simulink model "ALL_JP360_DBW_V6_5_1103"  (R2022a)
settings: Solver=FixedStepAuto  StartTime=0.0  StopTime=inf  FixedStep=0.01  RelTol=1e-3  EnableMultiTasking=on
model workspace (MAT data in the model file):
  g = 9.8
undefined symbols (not defined in the file or in its folder): canChannel, delta_v_p, IPM_Line_C0, IPM_Line_C1, IPM_Line_C2, IPM_Line_C3, M, M_p, MRR_ObjDistX, MRR_ObjDistY, MRR_ObjFusionCamID, MRR_ObjFusionSig, MRR_ObjID, MRR_ObjRelVelX, MRR_ObjRelVelY, MRR_ObjType, MRR_ObjUpdFlg, none, obj_vaild, untracktime, V, videoinput
libraries: canfdmsglib x230, canfdlib x76, slpidlib x24, simulink x18, dspstat3 x14, ctrlSharedLib x1, simulink_extras x1, imaqlib x1, realtime_pacer_lib x1, dspvision x1, visionsinks x1
(part 12 of 55)

== system ALL_JP360_DBW_V6_5_1103/MsgFromCAN/CCAN_ADCU_MsgFromCAN/CCAN_ADCU_SWM_Body_0x31A ==
  CCAN_ADCU_SWM_Body_0x31AFromInData : Inport  OutDataTypeStr=Bus:CAN_FD_MESSAGE_BUS
  Bus Creator : BusCreator  Inputs=28  OutDataTypeStr=Bus:CCAN_ADCU_SWM_Body_0x31A  NonVirtualBus=on
  CAN FD Unpack : canfdmsglib/CAN FD Unpack  CANdbFile=HiFire_JPT360_CCAN_Matrix_CAN_V1.72_VP_ADCU.dbc  MsgList=(none)  MsgName=SWM_Body_0x31A  ProtocolMode=CAN FD  MsgIDType=Standard (11-bit identifier)  MsgIdentifier=794  MsgLength=8  SignalInfo={'Checksum_0x31A','56','8','BE','unsigned','Standard','0','1','0','0','255';'RollingCounter_0x31A','48','4','BE','unsigned','Standard','0','1','0','0','15';'SWM_FWasherSts','4','2','BE','unsigned','Standard','0','1','0','0','3';'SWM_FlashLightSts','8','2','BE','unsigned','Standard','0','1','0','0','3';'SWM_FrontFogLight','18','2','BE','unsigned','Standard','0','1','0','0','3';'SWM_FrontWipingMode','10','3','BE','unsigned','Standard','0','1','0','0','7';'SWM_HeadLamp','29','3','BE','unsigned','Standard','0','1','0','0','3';'SWM_HighBeam','0','2','BE','unsigned','Standard','0','1','0','0','3';'SWM_LampLimpHomeSts','3','1','BE','unsigned','Standard','0','1','0','0','1';'SWM_Menu_Confirm','54','2','BE','unsigned','Standard','0','1','0','0','3';'SWM_Menu_Down','44','2','BE','unsigned','Standard','0','1','0','0','3';'SWM_Menu_Left','42','2','BE','unsigned','Standard','0','1','0','0','3';'SWM_Menu_Return','52','2','BE','unsigned','Standard','0','1','0','0','3';'SWM_Menu_Right','40','2','BE','unsigned','Standard','0','1','0','0','3';'SWM_Menu_Up','46','2','BE','unsigned','Standard','0','1','0','0','3';'SWM_Mute','38','2','BE','unsigned','Standard','0','1','0','0','3';'SWM_Next_Song','32','2','BE','unsigned','Standard','0','1','0','0','3';'SWM_Phone','36','2','BE','unsigned','Standard','0','1','0','0','3';'SWM_Previous_Song','34','2','BE','unsigned','Standard','0','1','0','0','3';'SWM_RWasherSts','6','2','BE','unsigned','Standard','0','1','0','0','3';'SWM_RearFogLight','16','2','BE','unsigned','Standard','0','1','0','0','3';'SWM_RearWipingMode','20','2','BE','unsigned','Standard','0','1','0','0','3';'SWM_TurnIndicationAct','22','2','BE','unsigned','Standard','0','1','0','0','3';'SWM_VOL_Minus','26','2','BE','unsigned','Standard','0','1','0','0','3';'SWM_VOL_Plus','24','2','BE','unsigned','Standard','0','1','0','0','3';'SWM_WasherLimpHomeSts','2','1','BE','unsigned','Standard','0','1','0','0','1';'SWM_Wechat','28','1','BE','unsigned','Standard','0','1','0','0','1';'SWM_WipingInterval_Sensitvity','13','3','BE','unsigned','Standard','0','1','0','0','7'}  IDPort=off  TimestampPort=off  ErrorPort=off  RemotePort=off  LengthPort=off  StatusPort=off  BRSPort=off  ESIPort=off  DLCPort=off  ApplyMinMax=off
      settings: SourceProductBaseCode=XP,ME,VN  DataFormat=CANdb specified signals
  Data Type Conversion1 : DataTypeConversion  OutDataTypeStr=uint8  SaturateOnIntegerOverflow=off  RndMeth=Floor
  Data Type Conversion{2..8,10..25,28} (24 alike) : DataTypeConversion  OutDataTypeStr=int8  SaturateOnIntegerOverflow=off  RndMeth=Floor
  Data Type Conversion26 : DataTypeConversion  OutDataTypeStr=boolean  SaturateOnIntegerOverflow=off  RndMeth=Floor
  Data Type Conversion27 : DataTypeConversion  OutDataTypeStr=boolean  SaturateOnIntegerOverflow=off  RndMeth=Floor
  Data Type Conversion9 : DataTypeConversion  OutDataTypeStr=boolean  SaturateOnIntegerOverflow=off  RndMeth=Floor
  CCAN_ADCU_SWM_Body_0x31AFromOutData : Outport  OutDataTypeStr=Bus:CCAN_ADCU_SWM_Body_0x31A
  wires:
  CAN FD Unpack/1 -> Data Type Conversion1/1
  CAN FD Unpack/2 -> Data Type Conversion2/1
  CAN FD Unpack/3 -> Data Type Conversion3/1
  CAN FD Unpack/4 -> Data Type Conversion4/1
  CAN FD Unpack/5 -> Data Type Conversion5/1
  CAN FD Unpack/6 -> Data Type Conversion6/1
  CAN FD Unpack/7 -> Data Type Conversion7/1
  CAN FD Unpack/8 -> Data Type Conversion8/1
  CAN FD Unpack/9 -> Data Type Conversion9/1
  CAN FD Unpack/10 -> Data Type Conversion10/1
  CAN FD Unpack/11 -> Data Type Conversion11/1
  CAN FD Unpack/12 -> Data Type Conversion12/1
  CAN FD Unpack/13 -> Data Type Conversion13/1
  CAN FD Unpack/14 -> Data Type Conversion14/1
  CAN FD Unpack/15 -> Data Type Conversion15/1
  CAN FD Unpack/16 -> Data Type Conversion16/1
  CAN FD Unpack/17 -> Data Type Conversion17/1
  CAN FD Unpack/18 -> Data Type Conversion18/1
  CAN FD Unpack/19 -> Data Type Conversion19/1
  CAN FD Unpack/20 -> Data Type Conversion20/1
  CAN FD Unpack/21 -> Data Type Conversion21/1
  CAN FD Unpack/22 -> Data Type Conversion22/1
  CAN FD Unpack/23 -> Data Type Conversion23/1
  CAN FD Unpack/24 -> Data Type Conversion24/1
  CAN FD Unpack/25 -> Data Type Conversion25/1
  CAN FD Unpack/26 -> Data Type Conversion26/1
  CAN FD Unpack/27 -> Data Type Conversion27/1
  CAN FD Unpack/28 -> Data Type Conversion28/1
  Data Type Conversion1/1 -> Bus Creator/1  "Checksum_0x31A"
  Data Type Conversion2/1 -> Bus Creator/2  "RollingCounter_0x31A"
  Data Type Conversion3/1 -> Bus Creator/3  "SWM_FWasherSts"
  Data Type Conversion4/1 -> Bus Creator/4  "SWM_FlashLightSts"
  Data Type Conversion5/1 -> Bus Creator/5  "SWM_FrontFogLight"
  Data Type Conversion6/1 -> Bus Creator/6  "SWM_FrontWipingMode"
  Data Type Conversion7/1 -> Bus Creator/7  "SWM_HeadLamp"
  Data Type Conversion8/1 -> Bus Creator/8  "SWM_HighBeam"
  Data Type Conversion9/1 -> Bus Creator/9  "SWM_LampLimpHomeSts"
  Data Type Conversion10/1 -> Bus Creator/10  "SWM_Menu_Confirm"
  Data Type Conversion11/1 -> Bus Creator/11  "SWM_Menu_Down"
  Data Type Conversion12/1 -> Bus Creator/12  "SWM_Menu_Left"
  Data Type Conversion13/1 -> Bus Creator/13  "SWM_Menu_Return"
  Data Type Conversion14/1 -> Bus Creator/14  "SWM_Menu_Right"
  Data Type Conversion15/1 -> Bus Creator/15  "SWM_Menu_Up"
  Data Type Conversion16/1 -> Bus Creator/16  "SWM_Mute"
  Data Type Conversion17/1 -> Bus Creator/17  "SWM_Next_Song"
  Data Type Conversion18/1 -> Bus Creator/18  "SWM_Phone"
  Data Type Conversion19/1 -> Bus Creator/19  "SWM_Previous_Song"
  Data Type Conversion20/1 -> Bus Creator/20  "SWM_RWasherSts"
  Data Type Conversion21/1 -> Bus Creator/21  "SWM_RearFogLight"
  Data Type Conversion22/1 -> Bus Creator/22  "SWM_RearWipingMode"
  Data Type Conversion23/1 -> Bus Creator/23  "SWM_TurnIndicationAct"
  Data Type Conversion24/1 -> Bus Creator/24  "SWM_VOL_Minus"
  Data Type Conversion25/1 -> Bus Creator/25  "SWM_VOL_Plus"
  Data Type Conversion26/1 -> Bus Creator/26  "SWM_WasherLimpHomeSts"
  Data Type Conversion27/1 -> Bus Creator/27  "SWM_Wechat"
  Data Type Conversion28/1 -> Bus Creator/28  "SWM_WipingInterval_Sensitvity"
  Bus Creator/1 -> CCAN_ADCU_SWM_Body_0x31AFromOutData/1  "CCAN_ADCU_SWM_Body_0x31AFromOutData"
  CCAN_ADCU_SWM_Body_0x31AFromInData/1 -> CAN FD Unpack/1  "CCAN_ADCU_SWM_Body_0x31AFromInData"

== system ALL_JP360_DBW_V6_5_1103/MsgFromCAN/CCAN_ADCU_MsgFromCAN/CCAN_ADCU_SWM_MRR_0x31B ==
  CCAN_ADCU_SWM_MRR_0x31BFromInData : Inport  OutDataTypeStr=Bus:CAN_FD_MESSAGE_BUS
  Bus Creator : BusCreator  Inputs=22  OutDataTypeStr=Bus:CCAN_ADCU_SWM_MRR_0x31B  NonVirtualBus=on
  CAN FD Unpack : canfdmsglib/CAN FD Unpack  CANdbFile=HiFire_JPT360_CCAN_Matrix_CAN_V1.72_VP_ADCU.dbc  MsgList=(none)  MsgName=SWM_MRR_0x31B  ProtocolMode=CAN FD  MsgIDType=Standard (11-bit identifier)  MsgIdentifier=795  MsgLength=8  SignalInfo={'BCM_CCO_Switch','20','1','BE','unsigned','Standard','0','1','0','0','1';'BCM_TAB_Switch','19','1','BE','unsigned','Standard','0','1','0','0','1';'Checksum_0x31B','56','8','BE','unsigned','Standard','0','1','0','0','255';'RollingCounter_0x31B','48','4','BE','unsigned','Standard','0','1','0','0','15';'SWM_ACCDeactivate','3','1','BE','unsigned','Standard','0','1','0','0','1';'SWM_ACCLimpHomeSts','11','1','BE','unsigned','Standard','0','1','0','0','1';'SWM_ACCResume','4','1','BE','unsigned','Standard','0','1','0','0','1';'SWM_ACCResume_Qt','7','1','BE','unsigned','Standard','0','1','0','0','1';'SWM_ACCSet','5','1','BE','unsigned','Standard','0','1','0','0','1';'SWM_ACCSwitch','12','1','BE','unsigned','Standard','0','1','0','0','1';'SWM_ACCtauGapSetMinus','15','1','BE','unsigned','Standard','0','1','0','0','1';'SWM_ACCtauGapSetPlus','0','1','BE','unsigned','Standard','0','1','0','0','1';'SWM_ACCvSetMinus','1','1','BE','unsigned','Standard','0','1','0','0','1';'SWM_ACCvSetPlus','2','1','BE','unsigned','Standard','0','1','0','0','1';'SWM_CCEnableSwitch','6','1','BE','unsigned','Standard','0','1','0','0','1';'SWM_ICorIVI','21','1','BE','unsigned','Standard','0','1','0','0','1';'SWM_LaneAssistSwitch','14','1','BE','unsigned','Standard','0','1','0','0','1';'SWM_MyButton','22','1','BE','unsigned','Standard','0','1','0','0','1';'SWM_ShiftPadFlt','23','1','BE','unsigned','Standard','0','1','0','0','1';'SWM_ShiftPadReqDown','9','1','BE','unsigned','Standard','0','1','0','0','1';'SWM_ShiftPadReqUp','10','1','BE','unsigned','Standard','0','1','0','0','1';'SWM_TJASwitch','8','1','BE','unsigned','Standard','0','1','0','0','1'}  IDPort=off  TimestampPort=off  ErrorPort=off  RemotePort=off  LengthPort=off  StatusPort=off  BRSPort=off  ESIPort=off  DLCPort=off  ApplyMinMax=off
      settings: SourceProductBaseCode=XP,ME,VN  DataFormat=CANdb specified signals
  Data Type Conversion{1..2,5..22} (20 alike) : DataTypeConversion  OutDataTypeStr=boolean  SaturateOnIntegerOverflow=off  RndMeth=Floor
  Data Type Conversion3 : DataTypeConversion  OutDataTypeStr=uint8  SaturateOnIntegerOverflow=off  RndMeth=Floor
  Data Type Conversion4 : DataTypeConversion  OutDataTypeStr=int8  SaturateOnIntegerOverflow=off  RndMeth=Floor
  CCAN_ADCU_SWM_MRR_0x31BFromOutData : Outport  OutDataTypeStr=Bus:CCAN_ADCU_SWM_MRR_0x31B
  wires:
  CAN FD Unpack/1 -> Data Type Conversion1/1
  CAN FD Unpack/2 -> Data Type Conversion2/1
  CAN FD Unpack/3 -> Data Type Conversion3/1
  CAN FD Unpack/4 -> Data Type Conversion4/1
  CAN FD Unpack/5 -> Data Type Conversion5/1
  CAN FD Unpack/6 -> Data Type Conversion6/1
  CAN FD Unpack/7 -> Data Type Conversion7/1
  CAN FD Unpack/8 -> Data Type Conversion8/1
  CAN FD Unpack/9 -> Data Type Conversion9/1
  CAN FD Unpack/10 -> Data Type Conversion10/1
  CAN FD Unpack/11 -> Data Type Conversion11/1
  CAN FD Unpack/12 -> Data Type Conversion12/1
  CAN FD Unpack/13 -> Data Type Conversion13/1
  CAN FD Unpack/14 -> Data Type Conversion14/1
  CAN FD Unpack/15 -> Data Type Conversion15/1
  CAN FD Unpack/16 -> Data Type Conversion16/1
  CAN FD Unpack/17 -> Data Type Conversion17/1
  CAN FD Unpack/18 -> Data Type Conversion18/1
  CAN FD Unpack/19 -> Data Type Conversion19/1
  CAN FD Unpack/20 -> Data Type Conversion20/1
  CAN FD Unpack/21 -> Data Type Conversion21/1
  CAN FD Unpack/22 -> Data Type Conversion22/1
  Data Type Conversion1/1 -> Bus Creator/1  "BCM_CCO_Switch"
  Data Type Conversion2/1 -> Bus Creator/2  "BCM_TAB_Switch"
  Data Type Conversion3/1 -> Bus Creator/3  "Checksum_0x31B"
  Data Type Conversion4/1 -> Bus Creator/4  "RollingCounter_0x31B"
  Data Type Conversion5/1 -> Bus Creator/5  "SWM_ACCDeactivate"
  Data Type Conversion6/1 -> Bus Creator/6  "SWM_ACCLimpHomeSts"
  Data Type Conversion7/1 -> Bus Creator/7  "SWM_ACCResume"
  Data Type Conversion8/1 -> Bus Creator/8  "SWM_ACCResume_Qt"
  Data Type Conversion9/1 -> Bus Creator/9  "SWM_ACCSet"
  Data Type Conversion10/1 -> Bus Creator/10  "SWM_ACCSwitch"
  Data Type Conversion11/1 -> Bus Creator/11  "SWM_ACCtauGapSetMinus"
  Data Type Conversion12/1 -> Bus Creator/12  "SWM_ACCtauGapSetPlus"
  Data Type Conversion13/1 -> Bus Creator/13  "SWM_ACCvSetMinus"
  Data Type Conversion14/1 -> Bus Creator/14  "SWM_ACCvSetPlus"
  Data Type Conversion15/1 -> Bus Creator/15  "SWM_CCEnableSwitch"
  Data Type Conversion16/1 -> Bus Creator/16  "SWM_ICorIVI"
  Data Type Conversion17/1 -> Bus Creator/17  "SWM_LaneAssistSwitch"
  Data Type Conversion18/1 -> Bus Creator/18  "SWM_MyButton"
  Data Type Conversion19/1 -> Bus Creator/19  "SWM_ShiftPadFlt"
  Data Type Conversion20/1 -> Bus Creator/20  "SWM_ShiftPadReqDown"
  Data Type Conversion21/1 -> Bus Creator/21  "SWM_ShiftPadReqUp"
  Data Type Conversion22/1 -> Bus Creator/22  "SWM_TJASwitch"
  Bus Creator/1 -> CCAN_ADCU_SWM_MRR_0x31BFromOutData/1  "CCAN_ADCU_SWM_MRR_0x31BFromOutData"
  CCAN_ADCU_SWM_MRR_0x31BFromInData/1 -> CAN FD Unpack/1  "CCAN_ADCU_SWM_MRR_0x31BFromInData"

== system ALL_JP360_DBW_V6_5_1103/MsgFromCAN/CCAN_ADCU_MsgFromCAN/CCAN_ADCU_Tester_DiagFuncReq ==
  CCAN_ADCU_Tester_DiagFuncReqFromInData : Inport  OutDataTypeStr=Bus:CAN_FD_MESSAGE_BUS
  Bus Creator : BusCreator  Inputs=1  OutDataTypeStr=Bus:CCAN_ADCU_Tester_DiagFuncReq  NonVirtualBus=on
  CAN FD Unpack : canfdmsglib/CAN FD Unpack  CANdbFile=HiFire_JPT360_CCAN_Matrix_CAN_V1.72_VP_ADCU.dbc  MsgList=(none)  MsgName=Tester_DiagFuncReq  ProtocolMode=CAN FD  MsgIDType=Standard (11-bit identifier)  MsgIdentifier=2015  MsgLength=8  SignalInfo={'DiagFuncReq','56','64','BE','unsigned','Standard','0','1','0','0','1.84467440737095e+19'}  IDPort=off  TimestampPort=off  ErrorPort=off  RemotePort=off  LengthPort=off  StatusPort=off  BRSPort=off  ESIPort=off  DLCPort=off  ApplyMinMax=off
      settings: SourceProductBaseCode=XP,ME,VN  DataFormat=CANdb specified signals
  Data Type Conversion1 : DataTypeConversion  OutDataTypeStr=uint64  SaturateOnIntegerOverflow=off  RndMeth=Floor
  CCAN_ADCU_Tester_DiagFuncReqFromOutData : Outport  OutDataTypeStr=Bus:CCAN_ADCU_Tester_DiagFuncReq
  wires:
  Data Type Conversion1/1 -> Bus Creator/1  "DiagFuncReq"
  Bus Creator/1 -> CCAN_ADCU_Tester_DiagFuncReqFromOutData/1  "CCAN_ADCU_Tester_DiagFuncReqFromOutData"
  CCAN_ADCU_Tester_DiagFuncReqFromInData/1 -> CAN FD Unpack/1  "CCAN_ADCU_Tester_DiagFuncReqFromInData"

== system ALL_JP360_DBW_V6_5_1103/MsgFromCAN/CCAN_ADCU_MsgFromCAN/CCAN_ADCU_Tester_DiagReqToADCU ==
  CCAN_ADCU_Tester_DiagReqToADCUFromInData : Inport  OutDataTypeStr=Bus:CAN_FD_MESSAGE_BUS
  Bus Creator : BusCreator  Inputs=1  OutDataTypeStr=Bus:CCAN_ADCU_Tester_DiagReqToADCU  NonVirtualBus=on
  CAN FD Unpack : canfdmsglib/CAN FD Unpack  CANdbFile=HiFire_JPT360_CCAN_Matrix_CAN_V1.72_VP_ADCU.dbc  MsgList=(none)  MsgName=Tester_DiagReqToADCU  ProtocolMode=CAN FD  MsgIDType=Standard (11-bit identifier)  MsgIdentifier=1809  MsgLength=8  SignalInfo={'DiagPhysReqToADCU','56','64','BE','unsigned','Standard','0','1','0','0','1.84467440737095e+19'}  IDPort=off  TimestampPort=off  ErrorPort=off  RemotePort=off  LengthPort=off  StatusPort=off  BRSPort=off  ESIPort=off  DLCPort=off  ApplyMinMax=off
      settings: SourceProductBaseCode=XP,ME,VN  DataFormat=CANdb specified signals
  Data Type Conversion1 : DataTypeConversion  OutDataTypeStr=uint64  SaturateOnIntegerOverflow=off  RndMeth=Floor
  CCAN_ADCU_Tester_DiagReqToADCUFromOutData : Outport  OutDataTypeStr=Bus:CCAN_ADCU_Tester_DiagReqToADCU
  wires:
  Data Type Conversion1/1 -> Bus Creator/1  "DiagPhysReqToADCU"
  Bus Creator/1 -> CCAN_ADCU_Tester_DiagReqToADCUFromOutData/1  "CCAN_ADCU_Tester_DiagReqToADCUFromOutData"
  CCAN_ADCU_Tester_DiagReqToADCUFromInData/1 -> CAN FD Unpack/1  "CCAN_ADCU_Tester_DiagReqToADCUFromInData"

== system ALL_JP360_DBW_V6_5_1103/MsgFromCAN/CCAN_GW_MsgFromCAN/CCAN_GW_ABS_Sts_0x221 ==
  CCAN_GW_ABS_Sts_0x221FromInData : Inport  OutDataTypeStr=Bus:CAN_FD_MESSAGE_BUS
  Bus Creator : BusCreator  Inputs=12  OutDataTypeStr=Bus:CCAN_GW_ABS_Sts_0x221  NonVirtualBus=on
  CAN FD Unpack : canfdmsglib/CAN FD Unpack  CANdbFile=HiFire_JPT360_CCAN_Matrix_CAN_V1.72_VP_ADCU.dbc  MsgList=(none)  MsgName=ABS_Sts_0x221  ProtocolMode=CAN FD  MsgIDType=Standard (11-bit identifier)  MsgIdentifier=545  MsgLength=8  SignalInfo={'ABS_AbsCtrlActv','39','1','BE','unsigned','Standard','0','1','0','0','1';'ABS_AbsFlgFlt','38','1','BE','unsigned','Standard','0','1','0','0','1';'ABS_EbdFlgFlt','37','1','BE','unsigned','Standard','0','1','0','0','1';'ABS_VehSpdDirection','36','1','BE','unsigned','Standard','0','1','0','0','1';'ABS_VehSpdLgt','40','12','BE','unsigned','Standard','0','0.05625','0','0','230.2875';'ABS_VehSpdLgtStatus','54','2','BE','unsigned','Standard','0','1','0','0','2';'ABS_WhlMilgFrntLe','8','16','BE','unsigned','Standard','0','1','0','0','65535';'ABS_WhlMilgFrntLeStatus','52','1','BE','unsigned','Standard','0','1','0','0','1';'ABS_WhlMilgFrntRi','24','16','BE','unsigned','Standard','0','1','0','0','65535';'ABS_WhlMilgFrntRiStatus','53','1','BE','unsigned','Standard','0','1','0','0','1';'Checksum_0x221','56','8','BE','unsigned','Standard','0','1','0','0','255';'RollingCounter_0x221','48','4','BE','unsigned','Standard','0','1','0','0','15'}  IDPort=off  TimestampPort=off  ErrorPort=off  RemotePort=off  LengthPort=off  StatusPort=off  BRSPort=off  ESIPort=off  DLCPort=off  ApplyMinMax=off
      settings: SourceProductBaseCode=XP,ME,VN  DataFormat=CANdb specified signals
  Data Type Conversion{1..4,8,10} (6 alike) : DataTypeConversion  OutDataTypeStr=boolean  SaturateOnIntegerOverflow=off  RndMeth=Floor
  Data Type Conversion11 : DataTypeConversion  OutDataTypeStr=uint8  SaturateOnIntegerOverflow=off  RndMeth=Floor
  Data Type Conversion12 : DataTypeConversion  OutDataTypeStr=int8  SaturateOnIntegerOverflow=off  RndMeth=Floor
  Data Type Conversion5 : DataTypeConversion  OutDataTypeStr=single  SaturateOnIntegerOverflow=off  RndMeth=Floor
  Data Type Conversion6 : DataTypeConversion  OutDataTypeStr=int8  SaturateOnIntegerOverflow=off  RndMeth=Floor
  Data Type Conversion7 : DataTypeConversion  OutDataTypeStr=uint16  SaturateOnIntegerOverflow=off  RndMeth=Floor
  Data Type Conversion9 : DataTypeConversion  OutDataTypeStr=uint16  SaturateOnIntegerOverflow=off  RndMeth=Floor
  CCAN_GW_ABS_Sts_0x221FromOutData : Outport  OutDataTypeStr=Bus:CCAN_GW_ABS_Sts_0x221
  wires:
  CAN FD Unpack/1 -> Data Type Conversion1/1
  CAN FD Unpack/2 -> Data Type Conversion2/1
  CAN FD Unpack/3 -> Data Type Conversion3/1
  CAN FD Unpack/4 -> Data Type Conversion4/1
  CAN FD Unpack/5 -> Data Type Conversion5/1
  CAN FD Unpack/6 -> Data Type Conversion6/1
  CAN FD Unpack/7 -> Data Type Conversion7/1
  CAN FD Unpack/8 -> Data Type Conversion8/1
  CAN FD Unpack/9 -> Data Type Conversion9/1
  CAN FD Unpack/10 -> Data Type Conversion10/1
  CAN FD Unpack/11 -> Data Type Conversion11/1
  CAN FD Unpack/12 -> Data Type Conversion12/1
  Data Type Conversion1/1 -> Bus Creator/1  "ABS_AbsCtrlActv"
  Data Type Conversion2/1 -> Bus Creator/2  "ABS_AbsFlgFlt"
  Data Type Conversion3/1 -> Bus Creator/3  "ABS_EbdFlgFlt"
  Data Type Conversion4/1 -> Bus Creator/4  "ABS_VehSpdDirection"
  Data Type Conversion5/1 -> Bus Creator/5  "ABS_VehSpdLgt"
  Data Type Conversion6/1 -> Bus Creator/6  "ABS_VehSpdLgtStatus"
  Data Type Conversion7/1 -> Bus Creator/7  "ABS_WhlMilgFrntLe"
  Data Type Conversion8/1 -> Bus Creator/8  "ABS_WhlMilgFrntLeStatus"
  Data Type Conversion9/1 -> Bus Creator/9  "ABS_WhlMilgFrntRi"
  Data Type Conversion10/1 -> Bus Creator/10  "ABS_WhlMilgFrntRiStatus"
  Data Type Conversion11/1 -> Bus Creator/11  "Checksum_0x221"
  Data Type Conversion12/1 -> Bus Creator/12  "RollingCounter_0x221"
  Bus Creator/1 -> CCAN_GW_ABS_Sts_0x221FromOutData/1  "CCAN_GW_ABS_Sts_0x221FromOutData"
  CCAN_GW_ABS_Sts_0x221FromInData/1 -> CAN FD Unpack/1  "CCAN_GW_ABS_Sts_0x221FromInData"

== system ALL_JP360_DBW_V6_5_1103/MsgFromCAN/CCAN_GW_MsgFromCAN/CCAN_GW_ABS_Vspeed_0x601 ==
  CCAN_GW_ABS_Vspeed_0x601FromInData : Inport  OutDataTypeStr=Bus:CAN_FD_MESSAGE_BUS
  Bus Creator : BusCreator  Inputs=2  OutDataTypeStr=Bus:CCAN_GW_ABS_Vspeed_0x601  NonVirtualBus=on
  CAN FD Unpack : canfdmsglib/CAN FD Unpack  CANdbFile=HiFire_JPT360_CCAN_Matrix_CAN_V1.72_VP_ADCU.dbc  MsgList=(none)  MsgName=ABS_Vspeed_0x601  ProtocolMode=CAN FD  MsgIDType=Standard (11-bit identifier)  MsgIdentifier=1537  MsgLength=8  SignalInfo={'ABS_VehSpd','8','16','BE','unsigned','Standard','0','0.0039062','0','0','250.996';'ABS_VehSpd_GB1','24','16','BE','unsigned','Standard','0','0.1','0','0','220'}  IDPort=off  TimestampPort=off  ErrorPort=off  RemotePort=off  LengthPort=off  StatusPort=off  BRSPort=off  ESIPort=off  DLCPort=off  ApplyMinMax=off
      settings: SourceProductBaseCode=XP,ME,VN  DataFormat=CANdb specified signals
  Data Type Conversion1 : DataTypeConversion  OutDataTypeStr=single  SaturateOnIntegerOverflow=off  RndMeth=Floor
  Data Type Conversion2 : DataTypeConversion  OutDataTypeStr=single  SaturateOnIntegerOverflow=off  RndMeth=Floor
  CCAN_GW_ABS_Vspeed_0x601FromOutData : Outport  OutDataTypeStr=Bus:CCAN_GW_ABS_Vspeed_0x601
  wires:
  CAN FD Unpack/1 -> Data Type Conversion1/1
  CAN FD Unpack/2 -> Data Type Conversion2/1
  Data Type Conversion1/1 -> Bus Creator/1  "ABS_VehSpd"
  Data Type Conversion2/1 -> Bus Creator/2  "ABS_VehSpd_GB1"
  Bus Creator/1 -> CCAN_GW_ABS_Vspeed_0x601FromOutData/1  "CCAN_GW_ABS_Vspeed_0x601FromOutData"
  CCAN_GW_ABS_Vspeed_0x601FromInData/1 -> CAN FD Unpack/1  "CCAN_GW_ABS_Vspeed_0x601FromInData"

== system ALL_JP360_DBW_V6_5_1103/MsgFromCAN/CCAN_GW_MsgFromCAN/CCAN_GW_ABS_WhlSpd_0x211 ==
  CCAN_GW_ABS_WhlSpd_0x211FromInData : Inport  OutDataTypeStr=Bus:CAN_FD_MESSAGE_BUS
  Bus Creator : BusCreator  Inputs=10  OutDataTypeStr=Bus:CCAN_GW_ABS_WhlSpd_0x211  NonVirtualBus=on
  CAN FD Unpack : canfdmsglib/CAN FD Unpack  CANdbFile=HiFire_JPT360_CCAN_Matrix_CAN_V1.72_VP_ADCU.dbc  MsgList=(none)  MsgName=ABS_WhlSpd_0x211  ProtocolMode=CAN FD  MsgIDType=Standard (11-bit identifier)  MsgIdentifier=529  MsgLength=8  SignalInfo={'ABS_WhlSpdFrntLe','12','12','BE','unsigned','Standard','0','0.05625','0','0','230.2875';'ABS_WhlSpdFrntLeStatus','55','1','BE','unsigned','Standard','0','1','0','0','1';'ABS_WhlSpdFrntRi','16','12','BE','unsigned','Standard','0','0.05625','0','0','230.2875';'ABS_WhlSpdFrntRiStatus','54','1','BE','unsigned','Standard','0','1','0','0','1';'ABS_WhlSpdReLe','36','12','BE','unsigned','Standard','0','0.05625','0','0','230.2875';'ABS_WhlSpdReLeStatus','53','1','BE','unsigned','Standard','0','1','0','0','1';'ABS_WhlSpdReRi','40','12','BE','unsigned','Standard','0','0.05625','0','0','230.2875';'ABS_WhlSpdReRiStatus','52','1','BE','unsigned','Standard','0','1','0','0','1';'Checksum_0x211','56','8','BE','unsigned','Standard','0','1','0','0','255';'RollingCounter_0x211','48','4','BE','unsigned','Standard','0','1','0','0','15'}  IDPort=off  TimestampPort=off  ErrorPort=off  RemotePort=off  LengthPort=off  StatusPort=off  BRSPort=off  ESIPort=off  DLCPort=off  ApplyMinMax=off
      settings: SourceProductBaseCode=XP,ME,VN  DataFormat=CANdb specified signals
  Data Type Conversion{1,3,5,7} (4 alike) : DataTypeConversion  OutDataTypeStr=single  SaturateOnIntegerOverflow=off  RndMeth=Floor
  Data Type Conversion10 : DataTypeConversion  OutDataTypeStr=int8  SaturateOnIntegerOverflow=off  RndMeth=Floor
  Data Type Conversion{2,4,6,8} (4 alike) : DataTypeConversion  OutDataTypeStr=boolean  SaturateOnIntegerOverflow=off  RndMeth=Floor
  Data Type Conversion9 : DataTypeConversion  OutDataTypeStr=uint8  SaturateOnIntegerOverflow=off  RndMeth=Floor
  CCAN_GW_ABS_WhlSpd_0x211FromOutData : Outport  OutDataTypeStr=Bus:CCAN_GW_ABS_WhlSpd_0x211
  wires:
  CAN FD Unpack/1 -> Data Type Conversion1/1
  CAN FD Unpack/2 -> Data Type Conversion2/1
  CAN FD Unpack/3 -> Data Type Conversion3/1
  CAN FD Unpack/4 -> Data Type Conversion4/1
  CAN FD Unpack/5 -> Data Type Conversion5/1
  CAN FD Unpack/6 -> Data Type Conversion6/1
  CAN FD Unpack/7 -> Data Type Conversion7/1
  CAN FD Unpack/8 -> Data Type Conversion8/1
  CAN FD Unpack/9 -> Data Type Conversion9/1
  CAN FD Unpack/10 -> Data Type Conversion10/1
  Data Type Conversion1/1 -> Bus Creator/1  "ABS_WhlSpdFrntLe"
  Data Type Conversion2/1 -> Bus Creator/2  "ABS_WhlSpdFrntLeStatus"
  Data Type Conversion3/1 -> Bus Creator/3  "ABS_WhlSpdFrntRi"
  Data Type Conversion4/1 -> Bus Creator/4  "ABS_WhlSpdFrntRiStatus"
  Data Type Conversion5/1 -> Bus Creator/5  "ABS_WhlSpdReLe"
  Data Type Conversion6/1 -> Bus Creator/6  "ABS_WhlSpdReLeStatus"
  Data Type Conversion7/1 -> Bus Creator/7  "ABS_WhlSpdReRi"
  Data Type Conversion8/1 -> Bus Creator/8  "ABS_WhlSpdReRiStatus"
  Data Type Conversion9/1 -> Bus Creator/9  "Checksum_0x211"
  Data Type Conversion10/1 -> Bus Creator/10  "RollingCounter_0x211"
  Bus Creator/1 -> CCAN_GW_ABS_WhlSpd_0x211FromOutData/1  "CCAN_GW_ABS_WhlSpd_0x211FromOutData"
  CCAN_GW_ABS_WhlSpd_0x211FromInData/1 -> CAN FD Unpack/1  "CCAN_GW_ABS_WhlSpd_0x211FromInData"

== system ALL_JP360_DBW_V6_5_1103/MsgFromCAN/CCAN_GW_MsgFromCAN/CCAN_GW_ADCU_0x538 ==
  CCAN_GW_ADCU_0x538FromInData : Inport  OutDataTypeStr=Bus:CAN_FD_MESSAGE_BUS
  Bus Creator : BusCreator  Inputs=2  OutDataTypeStr=Bus:CCAN_GW_ADCU_0x538  NonVirtualBus=on
  CAN FD Unpack : canfdmsglib/CAN FD Unpack  CANdbFile=HiFire_JPT360_CCAN_Matrix_CAN_V1.72_VP_ADCU.dbc  MsgList=(none)  MsgName=ADCU_0x538  ProtocolMode=CAN FD  MsgIDType=Standard (11-bit identifier)  MsgIdentifier=1336  MsgLength=8  SignalInfo={'ADCU_state','6','2','BE','unsigned','Standard','0','1','0','0','3';'BSD_FCTB_State','0','1','BE','unsigned','Standard','0','1','0','0','1'}  IDPort=off  TimestampPort=off  ErrorPort=off  RemotePort=off  LengthPort=off  StatusPort=off  BRSPort=off  ESIPort=off  DLCPort=off  ApplyMinMax=off
      settings: SourceProductBaseCode=XP,ME,VN  DataFormat=CANdb specified signals
  Data Type Conversion1 : DataTypeConversion  OutDataTypeStr=int8  SaturateOnIntegerOverflow=off  RndMeth=Floor
  Data Type Conversion2 : DataTypeConversion  OutDataTypeStr=boolean  SaturateOnIntegerOverflow=off  RndMeth=Floor
  CCAN_GW_ADCU_0x538FromOutData : Outport  OutDataTypeStr=Bus:CCAN_GW_ADCU_0x538
  wires:
  CAN FD Unpack/1 -> Data Type Conversion1/1
  CAN FD Unpack/2 -> Data Type Conversion2/1
  Data Type Conversion1/1 -> Bus Creator/1  "ADCU_state"
  Data Type Conversion2/1 -> Bus Creator/2  "BSD_FCTB_State"
  Bus Creator/1 -> CCAN_GW_ADCU_0x538FromOutData/1  "CCAN_GW_ADCU_0x538FromOutData"
  CCAN_GW_ADCU_0x538FromInData/1 -> CAN FD Unpack/1  "CCAN_GW_ADCU_0x538FromInData"

== system ALL_JP360_DBW_V6_5_1103/MsgFromCAN/CCAN_GW_MsgFromCAN/CCAN_GW_ADCU_CanTSyn_0x570 ==
  CCAN_GW_ADCU_CanTSyn_0x570FromInData : Inport  OutDataTypeStr=Bus:CAN_FD_MESSAGE_BUS
  Bus Creator : BusCreator  Inputs=1  OutDataTypeStr=Bus:CCAN_GW_ADCU_CanTSyn_0x570  NonVirtualBus=on
  CAN FD Unpack : canfdmsglib/CAN FD Unpack  CANdbFile=HiFire_JPT360_CCAN_Matrix_CAN_V1.72_VP_ADCU.dbc  MsgList=(none)  MsgName=ADCU_CanTSyn_0x570  ProtocolMode=CAN FD  MsgIDType=Standard (11-bit identifier)  MsgIdentifier=1392  MsgLength=8  SignalInfo={'CanTSyn','56','64','BE','unsigned','Standard','0','1','0','0','1.84467440737095e+19'}  IDPort=off  TimestampPort=off  ErrorPort=off  RemotePort=off  LengthPort=off  StatusPort=off  BRSPort=off  ESIPort=off  DLCPort=off  ApplyMinMax=off
      settings: SourceProductBaseCode=XP,ME,VN  DataFormat=CANdb specified signals
  Data Type Conversion1 : DataTypeConversion  OutDataTypeStr=uint64  SaturateOnIntegerOverflow=off  RndMeth=Floor
  CCAN_GW_ADCU_CanTSyn_0x570FromOutData : Outport  OutDataTypeStr=Bus:CCAN_GW_ADCU_CanTSyn_0x570
  wires:
  Data Type Conversion1/1 -> Bus Creator/1  "CanTSyn"
  Bus Creator/1 -> CCAN_GW_ADCU_CanTSyn_0x570FromOutData/1  "CCAN_GW_ADCU_CanTSyn_0x570FromOutData"
  CCAN_GW_ADCU_CanTSyn_0x570FromInData/1 -> CAN FD Unpack/1  "CCAN_GW_ADCU_CanTSyn_0x570FromInData"

== system ALL_JP360_DBW_V6_5_1103/MsgFromCAN/CCAN_GW_MsgFromCAN/CCAN_GW_BSD_0x275 ==
  CCAN_GW_BSD_0x275FromInData : Inport  OutDataTypeStr=Bus:CAN_FD_MESSAGE_BUS
  Bus Creator : BusCreator  Inputs=24  OutDataTypeStr=Bus:CCAN_GW_BSD_0x275  NonVirtualBus=on
  CAN FD Unpack : canfdmsglib/CAN FD Unpack  CANdbFile=HiFire_JPT360_CCAN_Matrix_CAN_V1.72_VP_ADCU.dbc  MsgList=(none)  MsgName=BSD_0x275  ProtocolMode=CAN FD  MsgIDType=Standard (11-bit identifier)  MsgIdentifier=629  MsgLength=8  SignalInfo={'BSDLCA_OFFTelltale','31','1','BE','unsigned','Standard','0','1','0','0','1';'BSD_AutoAlignmentFlag','8','2','BE','unsigned','Standard','0','1','0','0','3';'BSD_BLIS_Active','10','2','BE','unsigned','Standard','0','1','0','0','3';'BSD_BLIS_display','12','4','BE','unsigned','Standard','0','1','0','0','15';'BSD_BSDLCA_State','28','1','BE','unsigned','Standard','0','1','0','0','1';'BSD_DOA_State','26','1','BE','unsigned','Standard','0','1','0','0','1';'BSD_DOA_warningReqLeftFront','20','2','BE','unsigned','Standard','0','1','0','0','3';'BSD_DOA_warningReqLeftRear','18','2','BE','unsigned','Standard','0','1','0','0','3';'BSD_DOA_warningReqRightFront','4','2','BE','unsigned','Standard','0','1','0','0','3';'BSD_DOA_warningReqRightRear','2','2','BE','unsigned','Standard','0','1','0','0','3';'BSD_ELKwarning_left','25','1','BE','unsigned','Standard','0','1','0','0','1';'BSD_ELKwarning_right','24','1','BE','unsigned','Standard','0','1','0','0','1';'BSD_LCA_warningReqLeft','16','2','BE','unsigned','Standard','0','1','0','0','3';'BSD_LCA_warningReqRight','0','2','BE','unsigned','Standard','0','1','0','0','3';'BSD_RCTA_State','27','1','BE','unsigned','Standard','0','1','0','0','1';'BSD_RCTA_warningReqLeft','22','2','BE','unsigned','Standard','0','1','0','0','3';'BSD_RCTA_warningReqRight','6','2','BE','unsigned','Standard','0','1','0','0','3';'BSD_RCW_State','43','1','BE','unsigned','Standard','0','1','0','0','1';'BSD_RCW_warningReq','45','2','BE','unsigned','Standard','0','1','0','0','3';'Checksum_0x275','56','8','BE','unsigned','Standard','0','1','0','0','255';'DOA_OFFTelltale','29','1','BE','unsigned','Standard','0','1','0','0','1';'RCTA_OFFTelltale','30','1','BE','unsigned','Standard','0','1','0','0','1';'RCW_OFFTelltale','44','1','BE','unsigned','Standard','0','1','0','0','1';'RollingCounter_0x275','48','4','BE','unsigned','Standard','0','1','0','0','15'}  IDPort=off  TimestampPort=off  ErrorPort=off  RemotePort=off  LengthPort=off  StatusPort=off  BRSPort=off  ESIPort=off  DLCPort=off  ApplyMinMax=off
      settings: SourceProductBaseCode=XP,ME,VN  DataFormat=CANdb specified signals
  Data Type Conversion{1,5..6,11..12,15,18,21..23} (10 alike) : DataTypeConversion  OutDataTypeStr=boolean  SaturateOnIntegerOverflow=off  RndMeth=Floor
  Data Type Conversion{2..4,7..10,13..14,16..17,19,24} (13 alike) : DataTypeConversion  OutDataTypeStr=int8  SaturateOnIntegerOverflow=off  RndMeth=Floor
  Data Type Conversion20 : DataTypeConversion  OutDataTypeStr=uint8  SaturateOnIntegerOverflow=off  RndMeth=Floor
  CCAN_GW_BSD_0x275FromOutData : Outport  OutDataTypeStr=Bus:CCAN_GW_BSD_0x275
  wires:
  CAN FD Unpack/1 -> Data Type Conversion1/1
  CAN FD Unpack/2 -> Data Type Conversion2/1
  CAN FD Unpack/3 -> Data Type Conversion3/1
  CAN FD Unpack/4 -> Data Type Conversion4/1
  CAN FD Unpack/5 -> Data Type Conversion5/1
  CAN FD Unpack/6 -> Data Type Conversion6/1
  CAN FD Unpack/7 -> Data Type Conversion7/1
  CAN FD Unpack/8 -> Data Type Conversion8/1
  CAN FD Unpack/9 -> Data Type Conversion9/1
  CAN FD Unpack/10 -> Data Type Conversion10/1
  CAN FD Unpack/11 -> Data Type Conversion11/1
  CAN FD Unpack/12 -> Data Type Conversion12/1
  CAN FD Unpack/13 -> Data Type Conversion13/1
  CAN FD Unpack/14 -> Data Type Conversion14/1
  CAN FD Unpack/15 -> Data Type Conversion15/1
  CAN FD Unpack/16 -> Data Type Conversion16/1
  CAN FD Unpack/17 -> Data Type Conversion17/1
  CAN FD Unpack/18 -> Data Type Conversion18/1
  CAN FD Unpack/19 -> Data Type Conversion19/1
  CAN FD Unpack/20 -> Data Type Conversion20/1
  CAN FD Unpack/21 -> Data Type Conversion21/1
  CAN FD Unpack/22 -> Data Type Conversion22/1
  CAN FD Unpack/23 -> Data Type Conversion23/1
  CAN FD Unpack/24 -> Data Type Conversion24/1
  Data Type Conversion1/1 -> Bus Creator/1  "BSDLCA_OFFTelltale"
  Data Type Conversion2/1 -> Bus Creator/2  "BSD_AutoAlignmentFlag"
  Data Type Conversion3/1 -> Bus Creator/3  "BSD_BLIS_Active"
  Data Type Conversion4/1 -> Bus Creator/4  "BSD_BLIS_display"
  Data Type Conversion5/1 -> Bus Creator/5  "BSD_BSDLCA_State"
  Data Type Conversion6/1 -> Bus Creator/6  "BSD_DOA_State"
  Data Type Conversion7/1 -> Bus Creator/7  "BSD_DOA_warningReqLeftFront"
  Data Type Conversion8/1 -> Bus Creator/8  "BSD_DOA_warningReqLeftRear"
  Data Type Conversion9/1 -> Bus Creator/9  "BSD_DOA_warningReqRightFront"
  Data Type Conversion10/1 -> Bus Creator/10  "BSD_DOA_warningReqRightRear"
  Data Type Conversion11/1 -> Bus Creator/11  "BSD_ELKwarning_left"
  Data Type Conversion12/1 -> Bus Creator/12  "BSD_ELKwarning_right"
  Data Type Conversion13/1 -> Bus Creator/13  "BSD_LCA_warningReqLeft"
  Data Type Conversion14/1 -> Bus Creator/14  "BSD_LCA_warningReqRight"
  Data Type Conversion15/1 -> Bus Creator/15  "BSD_RCTA_State"
  Data Type Conversion16/1 -> Bus Creator/16  "BSD_RCTA_warningReqLeft"
  Data Type Conversion17/1 -> Bus Creator/17  "BSD_RCTA_warningReqRight"
  Data Type Conversion18/1 -> Bus Creator/18  "BSD_RCW_State"
  Data Type Conversion19/1 -> Bus Creator/19  "BSD_RCW_warningReq"
  Data Type Conversion20/1 -> Bus Creator/20  "Checksum_0x275"
  Data Type Conversion21/1 -> Bus Creator/21  "DOA_OFFTelltale"
  Data Type Conversion22/1 -> Bus Creator/22  "RCTA_OFFTelltale"
  Data Type Conversion23/1 -> Bus Creator/23  "RCW_OFFTelltale"
  Data Type Conversion24/1 -> Bus Creator/24  "RollingCounter_0x275"
  Bus Creator/1 -> CCAN_GW_BSD_0x275FromOutData/1  "CCAN_GW_BSD_0x275FromOutData"
  CCAN_GW_BSD_0x275FromInData/1 -> CAN FD Unpack/1  "CCAN_GW_BSD_0x275FromInData"

== system ALL_JP360_DBW_V6_5_1103/MsgFromCAN/CCAN_GW_MsgFromCAN/CCAN_GW_EPS_0x260 ==
  CCAN_GW_EPS_0x260FromInData : Inport  OutDataTypeStr=Bus:CAN_FD_MESSAGE_BUS
  Bus Creator : BusCreator  Inputs=21  OutDataTypeStr=Bus:CCAN_GW_EPS_0x260  NonVirtualBus=on
  CAN FD Unpack : canfdmsglib/CAN FD Unpack  CANdbFile=HiFire_JPT360_CCAN_Matrix_CAN_V1.72_VP_ADCU.dbc  MsgList=(none)  MsgName=EPS_0x260  ProtocolMode=CAN FD  MsgIDType=Standard (11-bit identifier)  MsgIdentifier=608  MsgLength=8  SignalInfo={'Checksum_0x260','56','8','BE','unsigned','Standard','0','1','0','0','255';'EPS_F_ECUTempValid','26','1','BE','unsigned','Standard','0','1','0','0','1';'EPS_F_LoadInfo','8','1','BE','unsigned','Standard','0','1','0','0','1';'EPS_N_ECUTemp','32','8','BE','unsigned','Standard','0','1','-70','-70','185';'EPS_N_LoadInfo','9','7','BE','unsigned','Standard','0','1','0','0','127';'EPS_N_PerformanceRedu','40','8','BE','unsigned','Standard','0','0.5','0','0','100';'EPS_SASIndexSts','54','1','BE','unsigned','Standard','0','1','0','0','1';'EPS_SASSoftLimitLeftFlg','2','2','BE','unsigned','Standard','0','1','0','0','3';'EPS_SASSoftLimitRightFlg','0','2','BE','unsigned','Standard','0','1','0','0','3';'EPS_S_SafeLampRed','7','1','BE','unsigned','Standard','0','1','0','0','1';'EPS_S_WarningLampYellow','6','1','BE','unsigned','Standard','0','1','0','0','1';'EPS_St_DTCFlag','5','1','BE','unsigned','Standard','0','1','0','0','1';'EPS_St_EmergencyCANInterface','19','1','BE','unsigned','Standard','0','1','0','0','1';'EPS_St_EmergencyECU','18','1','BE','unsigned','Standard','0','1','0','0','1';'EPS_St_EmergencyMotor','17','1','BE','unsigned','Standard','0','1','0','0','1';'EPS_St_EmergencyOverTemp','21','1','BE','unsigned','Standard','0','1','0','0','1';'EPS_St_EmergencyOverVoltage','22','1','BE','unsigned','Standard','0','1','0','0','1';'EPS_St_EmergencyPowerLimit','16','1','BE','unsigned','Standard','0','1','0','0','1';'EPS_St_EmergencySensor','20','1','BE','unsigned','Standard','0','1','0','0','1';'EPS_St_EmergencyUnderVoltage','23','1','BE','unsigned','Standard','0','1','0','0','1';'RollingCounter_0x260','48','4','BE','unsigned','Standard','0','1','0','0','15'}  IDPort=off  TimestampPort=off  ErrorPort=off  RemotePort=off  LengthPort=off  StatusPort=off  BRSPort=off  ESIPort=off  DLCPort=off  ApplyMinMax=off
      settings: SourceProductBaseCode=XP,ME,VN  DataFormat=CANdb specified signals
  Data Type Conversion1 : DataTypeConversion  OutDataTypeStr=uint8  SaturateOnIntegerOverflow=off  RndMeth=Floor
  Data Type Conversion{2..3,7,10..20} (14 alike) : DataTypeConversion  OutDataTypeStr=boolean  SaturateOnIntegerOverflow=off  RndMeth=Floor
  Data Type Conversion{5,8..9,21} (4 alike) : DataTypeConversion  OutDataTypeStr=int8  SaturateOnIntegerOverflow=off  RndMeth=Floor
  Data Type Conversion4 : DataTypeConversion  OutDataTypeStr=int16  SaturateOnIntegerOverflow=off  RndMeth=Floor
  Data Type Conversion6 : DataTypeConversion  OutDataTypeStr=single  SaturateOnIntegerOverflow=off  RndMeth=Floor
  CCAN_GW_EPS_0x260FromOutData : Outport  OutDataTypeStr=Bus:CCAN_GW_EPS_0x260
  wires:
  CAN FD Unpack/1 -> Data Type Conversion1/1
  CAN FD Unpack/2 -> Data Type Conversion2/1
  CAN FD Unpack/3 -> Data Type Conversion3/1
  CAN FD Unpack/4 -> Data Type Conversion4/1
  CAN FD Unpack/5 -> Data Type Conversion5/1
  CAN FD Unpack/6 -> Data Type Conversion6/1
  CAN FD Unpack/7 -> Data Type Conversion7/1
  CAN FD Unpack/8 -> Data Type Conversion8/1
  CAN FD Unpack/9 -> Data Type Conversion9/1
  CAN FD Unpack/10 -> Data Type Conversion10/1
  CAN FD Unpack/11 -> Data Type Conversion11/1
  CAN FD Unpack/12 -> Data Type Conversion12/1
  CAN FD Unpack/13 -> Data Type Conversion13/1
  CAN FD Unpack/14 -> Data Type Conversion14/1
  CAN FD Unpack/15 -> Data Type Conversion15/1
  CAN FD Unpack/16 -> Data Type Conversion16/1
  CAN FD Unpack/17 -> Data Type Conversion17/1
  CAN FD Unpack/18 -> Data Type Conversion18/1
  CAN FD Unpack/19 -> Data Type Conversion19/1
  CAN FD Unpack/20 -> Data Type Conversion20/1
  CAN FD Unpack/21 -> Data Type Conversion21/1
  Data Type Conversion1/1 -> Bus Creator/1  "Checksum_0x260"
  Data Type Conversion2/1 -> Bus Creator/2  "EPS_F_ECUTempValid"
  Data Type Conversion3/1 -> Bus Creator/3  "EPS_F_LoadInfo"
  Data Type Conversion4/1 -> Bus Creator/4  "EPS_N_ECUTemp"
  Data Type Conversion5/1 -> Bus Creator/5  "EPS_N_LoadInfo"
  Data Type Conversion6/1 -> Bus Creator/6  "EPS_N_PerformanceRedu"
  Data Type Conversion7/1 -> Bus Creator/7  "EPS_SASIndexSts"
  Data Type Conversion8/1 -> Bus Creator/8  "EPS_SASSoftLimitLeftFlg"
  Data Type Conversion9/1 -> Bus Creator/9  "EPS_SASSoftLimitRightFlg"
  Data Type Conversion10/1 -> Bus Creator/10  "EPS_S_SafeLampRed"
  Data Type Conversion11/1 -> Bus Creator/11  "EPS_S_WarningLampYellow"
  Data Type Conversion12/1 -> Bus Creator/12  "EPS_St_DTCFlag"
  Data Type Conversion13/1 -> Bus Creator/13  "EPS_St_EmergencyCANInterface"
  Data Type Conversion14/1 -> Bus Creator/14  "EPS_St_EmergencyECU"
  Data Type Conversion15/1 -> Bus Creator/15  "EPS_St_EmergencyMotor"
  Data Type Conversion16/1 -> Bus Creator/16  "EPS_St_EmergencyOverTemp"
  Data Type Conversion17/1 -> Bus Creator/17  "EPS_St_EmergencyOverVoltage"
  Data Type Conversion18/1 -> Bus Creator/18  "EPS_St_EmergencyPowerLimit"
  Data Type Conversion19/1 -> Bus Creator/19  "EPS_St_EmergencySensor"
  Data Type Conversion20/1 -> Bus Creator/20  "EPS_St_EmergencyUnderVoltage"
  Data Type Conversion21/1 -> Bus Creator/21  "RollingCounter_0x260"
  Bus Creator/1 -> CCAN_GW_EPS_0x260FromOutData/1  "CCAN_GW_EPS_0x260FromOutData"
  CCAN_GW_EPS_0x260FromInData/1 -> CAN FD Unpack/1  "CCAN_GW_EPS_0x260FromInData"

== system ALL_JP360_DBW_V6_5_1103/MsgFromCAN/CCAN_GW_MsgFromCAN/CCAN_GW_EPS_Advanced_0x176 ==
  CCAN_GW_EPS_Advanced_0x176FromInData : Inport  OutDataTypeStr=Bus:CAN_FD_MESSAGE_BUS
  Bus Creator : BusCreator  Inputs=12  OutDataTypeStr=Bus:CCAN_GW_EPS_Advanced_0x176  NonVirtualBus=on
  CAN FD Unpack : canfdmsglib/CAN FD Unpack  CANdbFile=HiFire_JPT360_CCAN_Matrix_CAN_V1.72_VP_ADCU.dbc  MsgList=(none)  MsgName=EPS_Advanced_0x176  ProtocolMode=CAN FD  MsgIDType=Standard (11-bit identifier)  MsgIdentifier=374  MsgLength=8  SignalInfo={'Checksum_0x176','56','8','BE','unsigned','Standard','0','1','0','0','255';'EPS_EPSPAMInh','32','8','BE','unsigned','Standard','0','1','0','0','255';'EPS_EPSPAMSts','52','4','BE','unsigned','Standard','0','1','0','0','15';'EPS_LDWControlStatus','27','2','BE','unsigned','Standard','0','1','0','0','3';'EPS_LKAControlStatus','30','2','BE','unsigned','Standard','0','1','0','0','3';'EPS_LKAResponseTorque','17','11','BE','unsigned','Standard','0','0.01','-10.24','-10.24','10.22';'EPS_LKAResponseTorqueValid','16','1','BE','unsigned','Standard','0','1','0','0','1';'EPS_PAM_SteeringSts','29','1','BE','unsigned','Standard','0','1','0','0','1';'EPS_PwrSteeringModeSts','25','2','BE','unsigned','Standard','0','1','0','0','3';'EPS_TorsionBarTorque','13','11','BE','unsigned','Standard','0','0.01','-10.24','-10.24','10.22';'EPS_TosionBarTorqueValid','12','1','BE','unsigned','Standard','0','1','0','0','1';'RollingCounter_0x176','48','4','BE','unsigned','Standard','0','1','0','0','15'}  IDPort=off  TimestampPort=off  ErrorPort=off  RemotePort=off  LengthPort=off  StatusPort=off  BRSPort=off  ESIPort=off  DLCPort=off  ApplyMinMax=off
      settings: SourceProductBaseCode=XP,ME,VN  DataFormat=CANdb specified signals
  Data Type Conversion1 : DataTypeConversion  OutDataTypeStr=uint8  SaturateOnIntegerOverflow=off  RndMeth=Floor
  Data Type Conversion10 : DataTypeConversion  OutDataTypeStr=single  SaturateOnIntegerOverflow=off  RndMeth=Floor
  Data Type Conversion11 : DataTypeConversion  OutDataTypeStr=boolean  SaturateOnIntegerOverflow=off  RndMeth=Floor
  Data Type Conversion{3..5,9,12} (5 alike) : DataTypeConversion  OutDataTypeStr=int8  SaturateOnIntegerOverflow=off  RndMeth=Floor
  Data Type Conversion2 : DataTypeConversion  OutDataTypeStr=uint8  SaturateOnIntegerOverflow=off  RndMeth=Floor
  Data Type Conversion6 : DataTypeConversion  OutDataTypeStr=single  SaturateOnIntegerOverflow=off  RndMeth=Floor
  Data Type Conversion7 : DataTypeConversion  OutDataTypeStr=boolean  SaturateOnIntegerOverflow=off  RndMeth=Floor
  Data Type Conversion8 : DataTypeConversion  OutDataTypeStr=boolean  SaturateOnIntegerOverflow=off  RndMeth=Floor
  CCAN_GW_EPS_Advanced_0x176FromOutData : Outport  OutDataTypeStr=Bus:CCAN_GW_EPS_Advanced_0x176
  wires:
  CAN FD Unpack/1 -> Data Type Conversion1/1
  CAN FD Unpack/2 -> Data Type Conversion2/1
  CAN FD Unpack/3 -> Data Type Conversion3/1
  CAN FD Unpack/4 -> Data Type Conversion4/1
  CAN FD Unpack/5 -> Data Type Conversion5/1
  CAN FD Unpack/6 -> Data Type Conversion6/1
  CAN FD Unpack/7 -> Data Type Conversion7/1
  CAN FD Unpack/8 -> Data Type Conversion8/1
  CAN FD Unpack/9 -> Data Type Conversion9/1
  CAN FD Unpack/10 -> Data Type Conversion10/1
  CAN FD Unpack/11 -> Data Type Conversion11/1
  CAN FD Unpack/12 -> Data Type Conversion12/1
  Data Type Conversion1/1 -> Bus Creator/1  "Checksum_0x176"
  Data Type Conversion2/1 -> Bus Creator/2  "EPS_EPSPAMInh"
  Data Type Conversion3/1 -> Bus Creator/3  "EPS_EPSPAMSts"
  Data Type Conversion4/1 -> Bus Creator/4  "EPS_LDWControlStatus"
  Data Type Conversion5/1 -> Bus Creator/5  "EPS_LKAControlStatus"
  Data Type Conversion6/1 -> Bus Creator/6  "EPS_LKAResponseTorque"
  Data Type Conversion7/1 -> Bus Creator/7  "EPS_LKAResponseTorqueValid"
  Data Type Conversion8/1 -> Bus Creator/8  "EPS_PAM_SteeringSts"
  Data Type Conversion9/1 -> Bus Creator/9  "EPS_PwrSteeringModeSts"
  Data Type Conversion10/1 -> Bus Creator/10  "EPS_TorsionBarTorque"
  Data Type Conversion11/1 -> Bus Creator/11  "EPS_TosionBarTorqueValid"
  Data Type Conversion12/1 -> Bus Creator/12  "RollingCounter_0x176"
  Bus Creator/1 -> CCAN_GW_EPS_Advanced_0x176FromOutData/1  "CCAN_GW_EPS_Advanced_0x176FromOutData"
  CCAN_GW_EPS_Advanced_0x176FromInData/1 -> CAN FD Unpack/1  "CCAN_GW_EPS_Advanced_0x176FromInData"

== system ALL_JP360_DBW_V6_5_1103/MsgFromCAN/CCAN_GW_MsgFromCAN/CCAN_GW_EPS_NM_0x5C2 ==
  CCAN_GW_EPS_NM_0x5C2FromInData : Inport  OutDataTypeStr=Bus:CAN_FD_MESSAGE_BUS
  Bus Creator : BusCreator  Inputs=12  OutDataTypeStr=Bus:CCAN_GW_EPS_NM_0x5C2  NonVirtualBus=on
  CAN FD Unpack : canfdmsglib/CAN FD Unpack  CANdbFile=HiFire_JPT360_CCAN_Matrix_CAN_V1.72_VP_ADCU.dbc  MsgList=(none)  MsgName=EPS_NM_0x5C2  ProtocolMode=CAN FD  MsgIDType=Standard (11-bit identifier)  MsgIdentifier=1474  MsgLength=8  SignalInfo={'EPSActiveWakeUpBit','12','1','BE','unsigned','Standard','0','1','0','0','1';'EPSDiagnosticWakeUp','18','1','BE','unsigned','Standard','0','1','0','0','1';'EPSInDiagnosticSessionKeepCANbusAwake','34','1','BE','unsigned','Standard','0','1','0','0','1';'EPSLocalConditionsActiveKeepCANbusAwake','35','1','BE','unsigned','Standard','0','1','0','0','1';'EPSLocalConditionsActiveWakeUp','19','1','BE','unsigned','Standard','0','1','0','0','1';'EPSNMDestAddr','0','8','BE','unsigned','Standard','0','1','0','0','255';'EPSNMWakeUp','16','1','BE','unsigned','Standard','0','1','0','0','1';'EPSNetworkManagementStatus','24','8','BE','unsigned','Standard','0','1','0','0','255';'EPSPowerSourceKeepCANbusAwake','33','1','BE','unsigned','Standard','0','1','0','0','1';'EPSPowerSourceWakeUp','17','1','BE','unsigned','Standard','0','1','0','0','1';'EPSRepeatMessageRequest','8','1','BE','unsigned','Standard','0','1','0','0','1';'EPSTimerDontTimeOutKeepCANbusAwake','32','1','BE','unsigned','Standard','0','1','0','0','1'}  IDPort=off  TimestampPort=off  ErrorPort=off  RemotePort=off  LengthPort=off  StatusPort=off  BRSPort=off  ESIPort=off  DLCPort=off  ApplyMinMax=off
      settings: SourceProductBaseCode=XP,ME,VN  DataFormat=CANdb specified signals
  Data Type Conversion{1..5,7,9..12} (10 alike) : DataTypeConversion  OutDataTypeStr=boolean  SaturateOnIntegerOverflow=off  RndMeth=Floor
  Data Type Conversion6 : DataTypeConversion  OutDataTypeStr=uint8  SaturateOnIntegerOverflow=off  RndMeth=Floor
  Data Type Conversion8 : DataTypeConversion  OutDataTypeStr=uint8  SaturateOnIntegerOverflow=off  RndMeth=Floor
  CCAN_GW_EPS_NM_0x5C2FromOutData : Outport  OutDataTypeStr=Bus:CCAN_GW_EPS_NM_0x5C2
  wires:
  CAN FD Unpack/1 -> Data Type Conversion1/1
  CAN FD Unpack/2 -> Data Type Conversion2/1
  CAN FD Unpack/3 -> Data Type Conversion3/1
  CAN FD Unpack/4 -> Data Type Conversion4/1
  CAN FD Unpack/5 -> Data Type Conversion5/1
  CAN FD Unpack/6 -> Data Type Conversion6/1
  CAN FD Unpack/7 -> Data Type Conversion7/1
  CAN FD Unpack/8 -> Data Type Conversion8/1
  CAN FD Unpack/9 -> Data Type Conversion9/1
  CAN FD Unpack/10 -> Data Type Conversion10/1
  CAN FD Unpack/11 -> Data Type Conversion11/1
  CAN FD Unpack/12 -> Data Type Conversion12/1
  Data Type Conversion1/1 -> Bus Creator/1  "EPSActiveWakeUpBit"
  Data Type Conversion2/1 -> Bus Creator/2  "EPSDiagnosticWakeUp"
  Data Type Conversion3/1 -> Bus Creator/3  "EPSInDiagnosticSessionKeepCANbusAwake"
  Data Type Conversion4/1 -> Bus Creator/4  "EPSLocalConditionsActiveKeepCANbusAwake"
  Data Type Conversion5/1 -> Bus Creator/5  "EPSLocalConditionsActiveWakeUp"
  Data Type Conversion6/1 -> Bus Creator/6  "EPSNMDestAddr"
  Data Type Conversion7/1 -> Bus Creator/7  "EPSNMWakeUp"
  Data Type Conversion8/1 -> Bus Creator/8  "EPSNetworkManagementStatus"
  Data Type Conversion9/1 -> Bus Creator/9  "EPSPowerSourceKeepCANbusAwake"
  Data Type Conversion10/1 -> Bus Creator/10  "EPSPowerSourceWakeUp"
  Data Type Conversion11/1 -> Bus Creator/11  "EPSRepeatMessageRequest"
  Data Type Conversion12/1 -> Bus Creator/12  "EPSTimerDontTimeOutKeepCANbusAwake"
  Bus Creator/1 -> CCAN_GW_EPS_NM_0x5C2FromOutData/1  "CCAN_GW_EPS_NM_0x5C2FromOutData"
  CCAN_GW_EPS_NM_0x5C2FromInData/1 -> CAN FD Unpack/1  "CCAN_GW_EPS_NM_0x5C2FromInData"
